simulink model "interactive_Example"  (R2014a)
settings: Solver=ode45  StartTime=0.0  StopTime=10.0  RelTol=1e-3
settings Model: Creator=Botao  LastModifiedBy=Botao

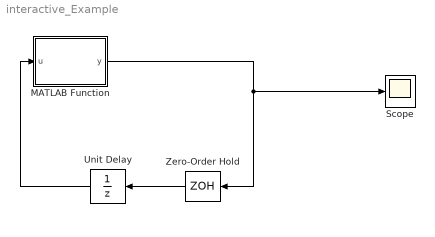
== system interactive_Example ==
  MATLAB Function : MATLAB Function  TreatAsAtomicUnit=on
  Scope : Scope
  Unit Delay : UnitDelay  SampleTime=-1
  Zero-Order Hold : ZeroOrderHold  SampleTime=-1
  wires:
  MATLAB Function/1(y) -> Zero-Order Hold/1, Scope/1
  Zero-Order Hold/1 -> Unit Delay/1
  Unit Delay/1 -> MATLAB Function/1(u)

== matlab function interactive_Example/MATLAB Function ==
  data: u input; y output
function y = fcn(u)
%#codegen

y=u+1;
